simulink model "fc_KTH_lib"  (Simulink 4.00)
settings: Solver=FixedStepDiscrete  StartTime=0.0  StopTime=5  RelTol=1e-3
undefined symbols (not defined in the file or in its folder): cell_const_F, cell_const_g, cell_const_jo, cell_const_LHV_H2, cell_const_Mair, cell_const_MH, cell_const_MW, cell_const_R2, cell_const_Voc, fan_cool, fc_act, fc_blower_rec_H2, fc_blowera, fc_cell_const_eta1, fc_cell_const_eta_DCDC, fc_cell_const_etablow, fc_cell_const_etagen, fc_cell_const_etapump, fc_cell_const_ex, fc_cell_const_kw, fc_cell_const_Nrad, fc_cell_const_U, fc_cell_dim_A, fc_cell_dim_tm, fc_cell_press_a, fc_cell_press_amb, fc_cell_press_an, fc_cell_press_blowa, fc_cell_press_blowr, fc_cell_press_c, fc_cell_press_hum, fc_cell_press_hyd, fc_cell_stack_dpipe, fc_cell_stack_dpipefc, fc_cell_stack_drad, fc_cell_stack_Lpipe, fc_cell_stack_Lpipefc, fc_cell_stack_Lrad, fc_cell_stack_N, fc_cell_stack_Pel, fc_cell_stoich_RHah, fc_cell_stoich_RHch, fc_cell_stoich_RHo, fc_cell_stoich_vH, fc_cell_stoich_vO, fc_cell_stoich_XON, fc_cell_temp_ah, fc_cell_temp_amb, fc_cell_temp_cell, fc_cell_temp_ch, fc_cell_temp_cond, fc_cell_temp_cool, fc_cell_temp_evap, fc_cell_temp_rad, fc_cell_temp_ref, fc_compressor, fc_conda, fc_condc, fc_coolstack, fc_current ... (+10)
(part 2 of 2)

== system fc_KTH_lib/PEM fuel cell system/Subsystem1/Anode init/Saturation pressure  anode humidifier ==
  note: Saturation pressure of water in the anode humidifier
      | NOTE: [bar]
      | Data from "Anlaggnings- och apparatteknik", Westerlund, T., Abo Akademi, Finland, 1998
  Anode humidifier temperature [C] : Constant  Value=fc_cell_temp_ah
  Anode humidifier temperature [C]1 : Constant  Value=fc_cell_temp_ah
  Constant : Constant  Value=11.78
  Constant1 : Constant  Value=99.64
  Constant2 : Constant  Value=230
  Math Function : Math  Operator=exp  OutputSignalType=auto
  Product : Product  Inputs=*/  Multiplication=Element-wise(.*)  SaturateOnIntegerOverflow=on
  Product1 : Product  Inputs=2  Multiplication=Element-wise(.*)  SaturateOnIntegerOverflow=on
  Sum : Sum  Inputs=|+-  SaturateOnIntegerOverflow=on
  Sum1 : Sum  Inputs=|++  SaturateOnIntegerOverflow=on
  psatah : Outport  Port=1
  wires:
  Anode humidifier temperature [C]/1 -> Sum/1
  Constant1/1 -> Sum/2
  Anode humidifier temperature [C]1/1 -> Sum1/1
  Constant2/1 -> Sum1/2
  Sum/1 -> Product/1
  Sum1/1 -> Product/2
  Constant/1 -> Product1/2
  Product/1 -> Product1/1
  Product1/1 -> Math Function/1
  Math Function/1 -> psatah/1

== system fc_KTH_lib/PEM fuel cell system/Subsystem1/Anode init/Subsystem2 ==
  note: Activity of water vapor
  XWaI [-] : Inport  Port=1  LatchInput=off
  psatah [bar] : Inport  Port=2  LatchInput=off
  Anode pressure : Constant  Value=fc_cell_press_a
  Product : Product  Inputs=2  Multiplication=Element-wise(.*)  SaturateOnIntegerOverflow=on
  Product1 : Product  Inputs=*/  Multiplication=Element-wise(.*)  SaturateOnIntegerOverflow=on
  a : Outport  Port=1
  wires:
  XWaI [-]/1 -> Product/1
  Anode pressure/1 -> Product/2
  Product/1 -> Product1/1
  psatah [bar]/1 -> Product1/2
  Product1/1 -> a/1

== system fc_KTH_lib/PEM fuel cell system/Fuel cell stack, Heat Generation/Heat/Latent heat [W]/Heat of condensation ==
  note: Temperature in Celsius (C)
      | Tref=25 C
  note: 45.07E3 - 41.9*Tcell + 3.44E-3*Tcell^2 + 2.54E-6*Tcell^3 -8.98E-10*Tcell^4
  note: Heat of condensation [J/mol]
  Cell temperature [C] : Constant  Value=fc_cell_temp_cell
  Constant1 : Constant  Value=3.44E-3
  Constant2 : Constant  Value=45.07E3
  Constant3 : Constant  Value=41.9
  Constant4 : Constant  Value=2.54E-6
  Constant5 : Constant  Value=3
  Constant6 : Constant  Value=4
  Constant7 : Constant  Value=8.98E-10
  Math Function : Math  Operator=square  OutputSignalType=auto
  Math Function1 : Math  Operator=pow  OutputSignalType=auto
  Math Function2 : Math  Operator=pow  OutputSignalType=auto
  Product{,1..3} (4 alike) : Product  Inputs=2  Multiplication=Element-wise(.*)  SaturateOnIntegerOverflow=on
  Sum : Sum  Inputs=|++  SaturateOnIntegerOverflow=on
  Sum1 : Sum  Inputs=|+-  SaturateOnIntegerOverflow=on
  Sum2 : Sum  Inputs=|++  SaturateOnIntegerOverflow=on
  Sum3 : Sum  Inputs=|+-  SaturateOnIntegerOverflow=on
  Hcond [J/mol] : Outport  Port=1
  wires:
  Constant3/1 -> Product/1
  Cell temperature [C]/1 -> Product/2, Math Function/1, Math Function1/1, Math Function2/1
  Product1/1 -> Sum/2
  Product/1 -> Sum1/2
  Constant2/1 -> Sum1/1
  Sum1/1 -> Sum/1
  Sum/1 -> Sum2/1
  Constant1/1 -> Product1/1
  Math Function/1 -> Product1/2
  Math Function1/1 -> Product2/2
  Constant4/1 -> Product2/1
  Product2/1 -> Sum2/2
  Sum2/1 -> Sum3/1
  Sum3/1 -> Hcond [J/mol]/1
  Math Function2/1 -> Product3/2
  Product3/1 -> Sum3/2
  Constant7/1 -> Product3/1
  Constant5/1 -> Math Function1/2
  Constant6/1 -> Math Function2/2

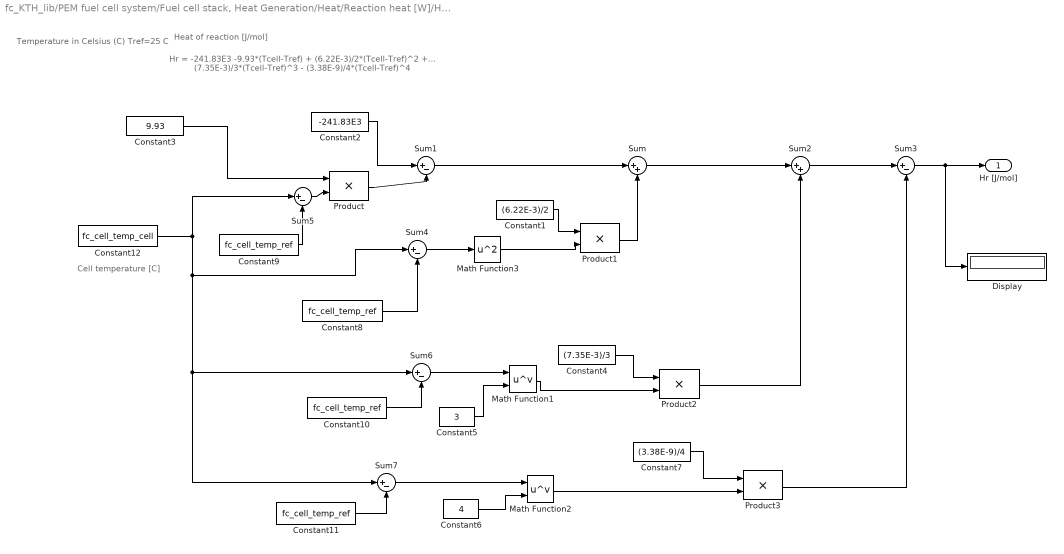
== system fc_KTH_lib/PEM fuel cell system/Fuel cell stack, Heat Generation/Heat/Reaction heat [W]/Heat of reaction ==
  note: Temperature in Celsius (C)
      | Tref=25 C
  note: Hr = -241.83E3 -9.93*(Tcell-Tref) + (6.22E-3)/2*(Tcell-Tref)^2 +...
      |   (7.35E-3)/3*(Tcell-Tref)^3 - (3.38E-9)/4*(Tcell-Tref)^4
  note: Heat of reaction [J/mol]
  note: Cell temperature [C]
  Constant1 : Constant  Value=(6.22E-3)/2
  Constant{8..11} (4 alike) : Constant  Value=fc_cell_temp_ref
  Constant12 : Constant  Value=fc_cell_temp_cell
  Constant2 : Constant  Value=-241.83E3
  Constant3 : Constant  Value=9.93
  Constant4 : Constant  Value=(7.35E-3)/3
  Constant5 : Constant  Value=3
  Constant6 : Constant  Value=4
  Constant7 : Constant  Value=(3.38E-9)/4
  Display : Display
      settings: Format=short  Decimation=12
  Math Function1 : Math  Operator=pow  OutputSignalType=auto
  Math Function2 : Math  Operator=pow  OutputSignalType=auto
  Math Function3 : Math  Operator=square  OutputSignalType=auto
  Product{,1..3} (4 alike) : Product  Inputs=2  Multiplication=Element-wise(.*)  SaturateOnIntegerOverflow=on
  Sum : Sum  Inputs=|++  SaturateOnIntegerOverflow=on
  Sum{1,3..7} (6 alike) : Sum  Inputs=|+-  SaturateOnIntegerOverflow=on
  Sum2 : Sum  Inputs=|++  SaturateOnIntegerOverflow=on
  Hr [J/mol] : Outport  Port=1
  wires:
  Constant3/1 -> Product/1
  Product1/1 -> Sum/2
  Product/1 -> Sum1/2
  Constant2/1 -> Sum1/1
  Sum1/1 -> Sum/1
  Sum/1 -> Sum2/1
  Constant1/1 -> Product1/1
  Math Function1/1 -> Product2/2
  Constant4/1 -> Product2/1
  Product2/1 -> Sum2/2
  Sum2/1 -> Sum3/1
  Sum3/1 -> Hr [J/mol]/1, Display/1
  Math Function2/1 -> Product3/2
  Product3/1 -> Sum3/2
  Constant7/1 -> Product3/1
  Constant5/1 -> Math Function1/2
  Constant6/1 -> Math Function2/2
  Constant8/1 -> Sum4/2
  Sum5/1 -> Product/2
  Constant9/1 -> Sum5/2
  Sum4/1 -> Math Function3/1
  Math Function3/1 -> Product1/2
  Constant10/1 -> Sum6/2
  Sum6/1 -> Math Function1/1
  Constant11/1 -> Sum7/2
  Sum7/1 -> Math Function2/1
  Constant12/1 -> Sum5/1, Sum4/1, Sum6/1, Sum7/1

== system fc_KTH_lib/PEM fuel cell system/Fuel cell stack, Heat Generation/Heat/Sensible heat [W]/Sensible heat in  ==
  note: Sensible heat in [W]
  note: Anode
  note: Cathode
  note: -------------------------------------------------------------------------------------------------------------------------------------------------------------------------------------------------------------------------------------------------------------------------------------------------------------------------------------------------------------------------------------------------------------------------------------------------------------------------------------------------------------------------------------------------------------------------------------------------------------------------------------------------------------------------------------------
  NinWa : Inport  Port=1  LatchInput=off
  NinHa : Inport  Port=2  LatchInput=off
  NinWc : Inport  Port=3  LatchInput=off
  NinO : Inport  Port=4  LatchInput=off
  NinN : Inport  Port=5  LatchInput=off
  "Enthalpy gaseous water, anode" : Subsystem
      settings: RTWFcnNameOpts=Auto  RTWFileNameOpts=Auto
  Enthalpy hydrogen in : Subsystem
      settings: RTWFcnNameOpts=Auto  RTWFileNameOpts=Auto
  Enthalpy nitrogen in : Subsystem
      settings: RTWFcnNameOpts=Auto  RTWFileNameOpts=Auto
  Enthalpy oxygen in : Subsystem
      settings: RTWFcnNameOpts=Auto  RTWFileNameOpts=Auto
  Product{,1..4} (5 alike) : Product  Inputs=2  Multiplication=Element-wise(.*)  SaturateOnIntegerOverflow=on
  Subsystem1 : Subsystem
      settings: RTWFcnNameOpts=Auto  RTWFileNameOpts=Auto
  Sum : Sum  Inputs=|++  SaturateOnIntegerOverflow=on
  Sum1 : Sum  Inputs=|++  SaturateOnIntegerOverflow=on
  Sum2 : Sum  Inputs=|++  SaturateOnIntegerOverflow=on
  sensina [W] : Outport  Port=1
  sensinc [W] : Outport  Port=2
  wires:
  NinHa/1 -> Product/1
  Enthalpy hydrogen in/1(h_Hin [J/mol]) -> Product/2
  Product/1 -> Sum/2
  NinWa/1 -> Product1/1
  Product1/1 -> Sum/1
  "Enthalpy gaseous water, anode"/1(h_Wgain [J/mol]) -> Product1/2
  NinWc/1 -> Product2/1
  Subsystem1/1(h_Wgcin [J/mol]) -> Product2/2
  Product2/1 -> Sum2/1
  NinO/1 -> Product3/1
  Enthalpy oxygen in/1(h_Oin [J/mol]) -> Product3/2
  Product3/1 -> Sum2/2
  Sum2/1 -> Sum1/1
  NinN/1 -> Product4/1
  Product4/1 -> Sum1/2
  Sum/1 -> sensina [W]/1
  Sum1/1 -> sensinc [W]/1
  Enthalpy nitrogen in/1(h_N [J/mol]) -> Product4/2

== system fc_KTH_lib/PEM fuel cell system/Fuel cell stack, Heat Generation/Heat/Sensible heat [W]/Sensible heat out ==
  note: Sensible heat out [W]
  note: Anode
  note: Cathode
  note: -------------------------------------------------------------------------------------------------------------------------------------------------------------------------------------------------------------------------------------------------------------------------------------------------------------------------------------------------------------------------------------------------------------------------------------------------------------------------------------------------------------------------------------------------------------------------------------------------------------------------------------------------------------------------------------------
  note: Enthalpy gaseous water, cathode
  NoutWag : Inport  Port=1  LatchInput=off
  NoutHa : Inport  Port=2  LatchInput=off
  NoutWcg : Inport  Port=3  LatchInput=off
  NoutO : Inport  Port=4  LatchInput=off
  NoutN : Inport  Port=5  LatchInput=off
  NoutWcl : Inport  Port=6  LatchInput=off
  "Enthalpy gaseous water, anode" : Subsystem
      settings: RTWFcnNameOpts=Auto  RTWFileNameOpts=Auto
  Enthalpy hydrogen in : Subsystem
      settings: RTWFcnNameOpts=Auto  RTWFileNameOpts=Auto
  Enthalpy nitrogen out : Subsystem
      settings: RTWFcnNameOpts=Auto  RTWFileNameOpts=Auto
  Enthalpy oxygen out : Subsystem
      settings: RTWFcnNameOpts=Auto  RTWFileNameOpts=Auto
  Product{,1..5} (6 alike) : Product  Inputs=2  Multiplication=Element-wise(.*)  SaturateOnIntegerOverflow=on
  Subsystem1 : Subsystem
      settings: RTWFcnNameOpts=Auto  RTWFileNameOpts=Auto
  Subsystem2 : Subsystem
      settings: RTWFcnNameOpts=Auto  RTWFileNameOpts=Auto
  Sum{,1..3} (4 alike) : Sum  Inputs=|++  SaturateOnIntegerOverflow=on
  sensouta [W] : Outport  Port=1
  sensoutc [W] : Outport  Port=2
  wires:
  NoutHa/1 -> Product/1
  Enthalpy hydrogen in/1(h_Hout [J/mol]) -> Product/2
  Product/1 -> Sum/2
  NoutWag/1 -> Product1/1
  Product1/1 -> Sum/1
  "Enthalpy gaseous water, anode"/1(h_Wgaout [J/mol]) -> Product1/2
  NoutWcg/1 -> Product2/1
  Subsystem1/1(h_Wgcout [J/mol]) -> Product2/2
  Product2/1 -> Sum2/1
  NoutO/1 -> Product3/1
  Enthalpy oxygen out/1(h_Oout [J/mol]) -> Product3/2
  Product3/1 -> Sum2/2
  Sum2/1 -> Sum1/1
  NoutN/1 -> Product4/1
  Product4/1 -> Sum1/2
  Sum/1 -> sensouta [W]/1
  Enthalpy nitrogen out/1(h_N [J/mol]) -> Product4/2
  Sum1/1 -> Sum3/1
  Sum3/1 -> sensoutc [W]/1
  Subsystem2/1(h_Wl [J/mol]) -> Product5/2
  Product5/1 -> Sum3/2
  NoutWcl/1 -> Product5/1

== system fc_KTH_lib/PEM fuel cell system/Humidifiers/Evapcooler/Ambient air/Humidity in air ==
  note: Humidity in air
  psat_air : Inport  Port=1  LatchInput=off
  Constant : Constant  Value=cell_const_MW
  Constant1 : Constant  Value=fc_cell_stoich_RHo
  Constant2 : Constant  Value=cell_const_Mair
  Constant3 : Constant  Value=fc_cell_press_amb
  Constant4 : Constant  Value=100
  Constant6 : Constant  Value=fc_cell_stoich_RHo
  Constant7 : Constant  Value=100
  Display : Display
      settings: Format=short
  Product : Product  Inputs=*/  Multiplication=Element-wise(.*)  SaturateOnIntegerOverflow=on
  Product1 : Product  Inputs=*/  Multiplication=Element-wise(.*)  SaturateOnIntegerOverflow=on
  Product2 : Product  Inputs=3  Multiplication=Element-wise(.*)  SaturateOnIntegerOverflow=on
  Product3 : Product  Inputs=*/  Multiplication=Element-wise(.*)  SaturateOnIntegerOverflow=on
  Product4 : Product  Inputs=2  Multiplication=Element-wise(.*)  SaturateOnIntegerOverflow=on
  Product5 : Product  Inputs=/*  Multiplication=Element-wise(.*)  SaturateOnIntegerOverflow=on
  Sum : Sum  Inputs=|+-  SaturateOnIntegerOverflow=on
  wires:
  Constant/1 -> Product/1
  Constant2/1 -> Product/2
  Constant1/1 -> Product1/1
  Constant4/1 -> Product1/2
  psat_air/1 -> Product2/1, Product4/2
  Product1/1 -> Product2/3
  Product/1 -> Product2/2
  Constant6/1 -> Product3/1
  Constant7/1 -> Product3/2
  Constant3/1 -> Sum/1
  Product3/1 -> Sum/2
  Sum/1 -> Product4/1
  Product2/1 -> Product5/2
  Product4/1 -> Product5/1
  Product5/1 -> Display/1

== system fc_KTH_lib/PEM fuel cell system/Humidifiers/Evapcooler/Ambient air/Saturation pressure ==
  note: Saturation pressure of water in the ambient air
      | NOTE: [bar]
      | Data from "Anlaggnings- och apparatteknik", Westerlund, T., Abo Akademi, Finland, 1998
  Ambient temperature [C] : Constant  Value=fc_cell_temp_amb
  Ambient temperature [C]1 : Constant  Value=fc_cell_temp_amb
  Constant : Constant  Value=11.78
  Constant1 : Constant  Value=99.64
  Constant2 : Constant  Value=230
  Math Function : Math  Operator=exp  OutputSignalType=auto
  Product : Product  Inputs=*/  Multiplication=Element-wise(.*)  SaturateOnIntegerOverflow=on
  Product1 : Product  Inputs=2  Multiplication=Element-wise(.*)  SaturateOnIntegerOverflow=on
  Sum : Sum  Inputs=|+-  SaturateOnIntegerOverflow=on
  Sum1 : Sum  Inputs=|++  SaturateOnIntegerOverflow=on
  psat_air : Outport  Port=1
  tag scope: psat_air=global
  wires:
  Ambient temperature [C]/1 -> Sum/1
  Constant1/1 -> Sum/2
  Ambient temperature [C]1/1 -> Sum1/1
  Constant2/1 -> Sum1/2
  Sum/1 -> Product/1
  Sum1/1 -> Product/2
  Constant/1 -> Product1/2
  Product/1 -> Product1/1
  Product1/1 -> Math Function/1
  Math Function/1 -> psat_air/1, [psat_air]

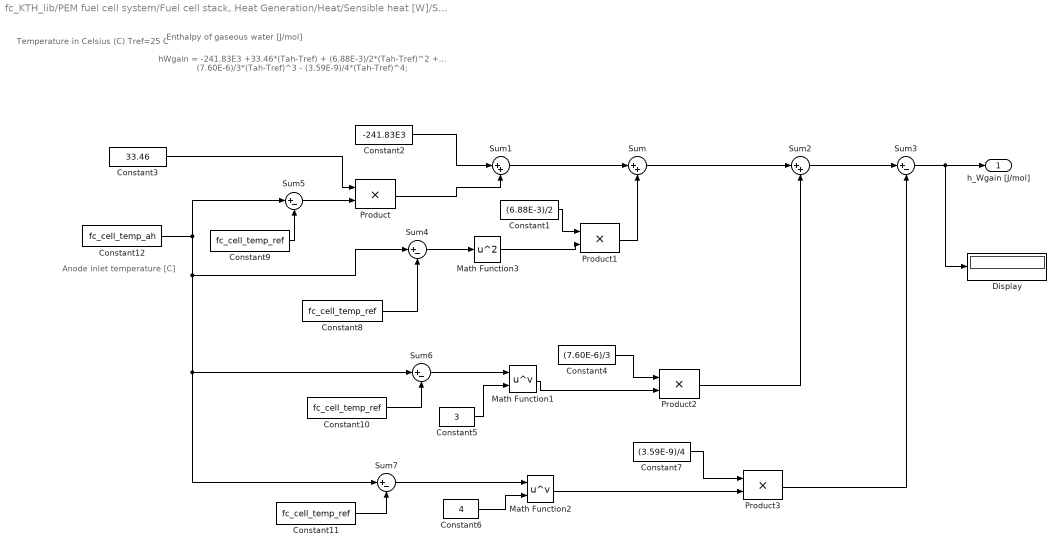
== system fc_KTH_lib/PEM fuel cell system/Fuel cell stack, Heat Generation/Heat/Sensible heat [W]/Sensible heat in /Enthalpy gaseous water, anode ==
  note: Temperature in Celsius (C)
      | Tref=25 C
  note: hWgain = -241.83E3 +33.46*(Tah-Tref) + (6.88E-3)/2*(Tah-Tref)^2 +...
      |    (7.60E-6)/3*(Tah-Tref)^3 - (3.59E-9)/4*(Tah-Tref)^4;
  note: Enthalpy of gaseous water [J/mol]
  note: Anode inlet temperature [C]
  Constant1 : Constant  Value=(6.88E-3)/2
  Constant{8..11} (4 alike) : Constant  Value=fc_cell_temp_ref
  Constant12 : Constant  Value=fc_cell_temp_ah
  Constant2 : Constant  Value=-241.83E3
  Constant3 : Constant  Value=33.46
  Constant4 : Constant  Value=(7.60E-6)/3
  Constant5 : Constant  Value=3
  Constant6 : Constant  Value=4
  Constant7 : Constant  Value=(3.59E-9)/4
  Display : Display
      settings: Format=short  Decimation=12
  Math Function1 : Math  Operator=pow  OutputSignalType=auto
  Math Function2 : Math  Operator=pow  OutputSignalType=auto
  Math Function3 : Math  Operator=square  OutputSignalType=auto
  Product{,1..3} (4 alike) : Product  Inputs=2  Multiplication=Element-wise(.*)  SaturateOnIntegerOverflow=on
  Sum : Sum  Inputs=|++  SaturateOnIntegerOverflow=on
  Sum1 : Sum  Inputs=|++  SaturateOnIntegerOverflow=on
  Sum2 : Sum  Inputs=|++  SaturateOnIntegerOverflow=on
  Sum{3..7} (5 alike) : Sum  Inputs=|+-  SaturateOnIntegerOverflow=on
  h_Wgain [J/mol] : Outport  Port=1
  wires:
  Constant3/1 -> Product/1
  Product1/1 -> Sum/2
  Sum/1 -> Sum2/1
  Constant1/1 -> Product1/1
  Math Function1/1 -> Product2/2
  Constant4/1 -> Product2/1
  Product2/1 -> Sum2/2
  Sum2/1 -> Sum3/1
  Sum3/1 -> h_Wgain [J/mol]/1, Display/1
  Math Function2/1 -> Product3/2
  Product3/1 -> Sum3/2
  Constant7/1 -> Product3/1
  Constant5/1 -> Math Function1/2
  Constant6/1 -> Math Function2/2
  Constant8/1 -> Sum4/2
  Sum5/1 -> Product/2
  Constant9/1 -> Sum5/2
  Sum4/1 -> Math Function3/1
  Math Function3/1 -> Product1/2
  Constant10/1 -> Sum6/2
  Sum6/1 -> Math Function1/1
  Constant11/1 -> Sum7/2
  Sum7/1 -> Math Function2/1
  Constant12/1 -> Sum5/1, Sum4/1, Sum6/1, Sum7/1
  Product/1 -> Sum1/2
  Sum1/1 -> Sum/1
  Constant2/1 -> Sum1/1

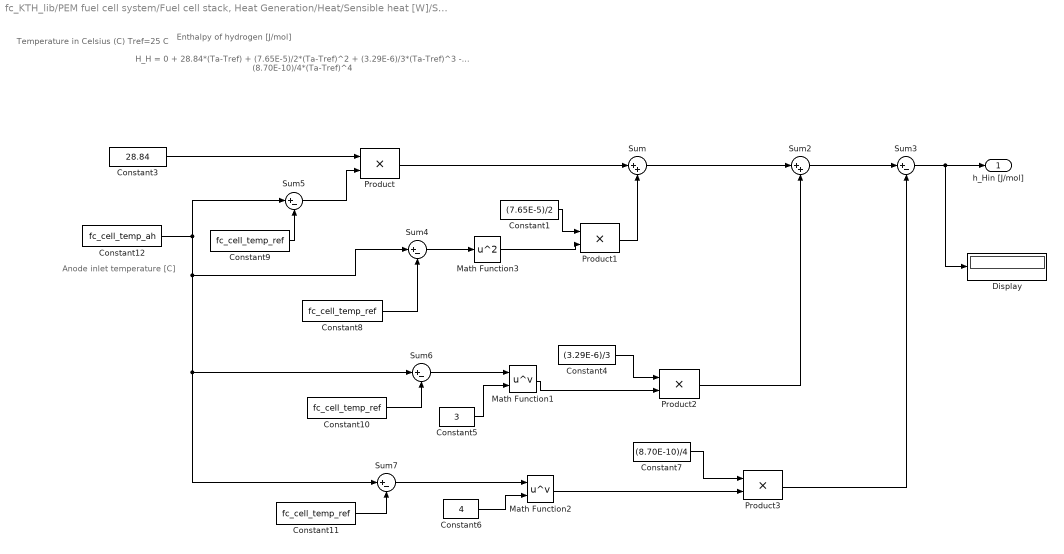
== system fc_KTH_lib/PEM fuel cell system/Fuel cell stack, Heat Generation/Heat/Sensible heat [W]/Sensible heat in /Enthalpy hydrogen in ==
  note: Temperature in Celsius (C)
      | Tref=25 C
  note: H_H = 0 + 28.84*(Ta-Tref) + (7.65E-5)/2*(Ta-Tref)^2 + (3.29E-6)/3*(Ta-Tref)^3 -...
      |    (8.70E-10)/4*(Ta-Tref)^4
  note: Enthalpy of hydrogen [J/mol]
  note: Anode inlet temperature [C]
  Constant1 : Constant  Value=(7.65E-5)/2
  Constant{8..11} (4 alike) : Constant  Value=fc_cell_temp_ref
  Constant12 : Constant  Value=fc_cell_temp_ah
  Constant3 : Constant  Value=28.84
  Constant4 : Constant  Value=(3.29E-6)/3
  Constant5 : Constant  Value=3
  Constant6 : Constant  Value=4
  Constant7 : Constant  Value=(8.70E-10)/4
  Display : Display
      settings: Format=short  Decimation=12
  Math Function1 : Math  Operator=pow  OutputSignalType=auto
  Math Function2 : Math  Operator=pow  OutputSignalType=auto
  Math Function3 : Math  Operator=square  OutputSignalType=auto
  Product{,1..3} (4 alike) : Product  Inputs=2  Multiplication=Element-wise(.*)  SaturateOnIntegerOverflow=on
  Sum : Sum  Inputs=|++  SaturateOnIntegerOverflow=on
  Sum2 : Sum  Inputs=|++  SaturateOnIntegerOverflow=on
  Sum{3..7} (5 alike) : Sum  Inputs=|+-  SaturateOnIntegerOverflow=on
  h_Hin [J/mol] : Outport  Port=1
  wires:
  Constant3/1 -> Product/1
  Product1/1 -> Sum/2
  Sum/1 -> Sum2/1
  Constant1/1 -> Product1/1
  Math Function1/1 -> Product2/2
  Constant4/1 -> Product2/1
  Product2/1 -> Sum2/2
  Sum2/1 -> Sum3/1
  Sum3/1 -> h_Hin [J/mol]/1, Display/1
  Math Function2/1 -> Product3/2
  Product3/1 -> Sum3/2
  Constant7/1 -> Product3/1
  Constant5/1 -> Math Function1/2
  Constant6/1 -> Math Function2/2
  Constant8/1 -> Sum4/2
  Sum5/1 -> Product/2
  Constant9/1 -> Sum5/2
  Sum4/1 -> Math Function3/1
  Math Function3/1 -> Product1/2
  Constant10/1 -> Sum6/2
  Sum6/1 -> Math Function1/1
  Constant11/1 -> Sum7/2
  Sum7/1 -> Math Function2/1
  Constant12/1 -> Sum5/1, Sum4/1, Sum6/1, Sum7/1
  Product/1 -> Sum/1

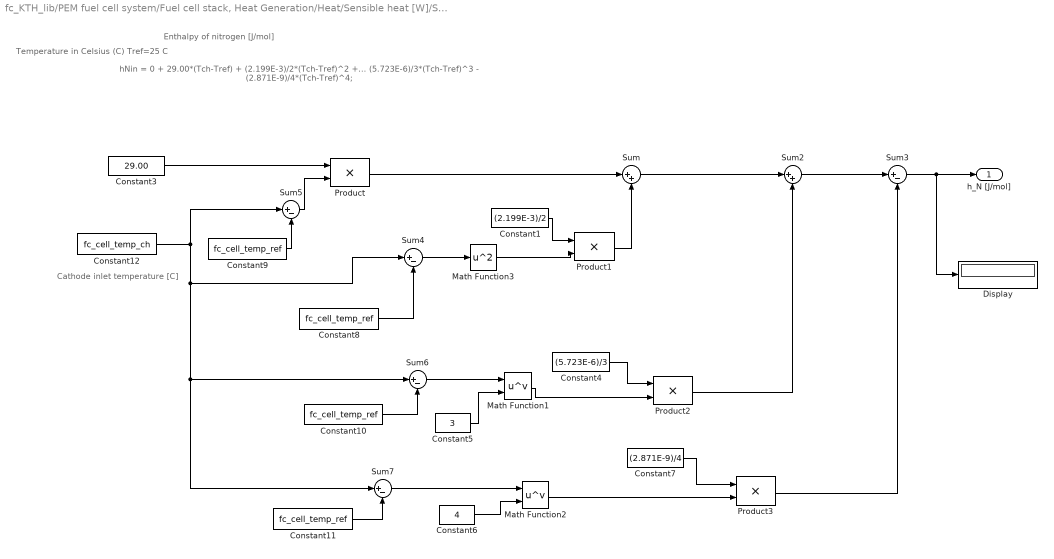
== system fc_KTH_lib/PEM fuel cell system/Fuel cell stack, Heat Generation/Heat/Sensible heat [W]/Sensible heat in /Enthalpy nitrogen in ==
  note: Temperature in Celsius (C)
      | Tref=25 C
  note: hNin = 0 + 29.00*(Tch-Tref) + (2.199E-3)/2*(Tch-Tref)^2 +...
      |    (5.723E-6)/3*(Tch-Tref)^3 - (2.871E-9)/4*(Tch-Tref)^4;
  note: Enthalpy of nitrogen [J/mol]
  note: Cathode inlet temperature [C]
  Constant1 : Constant  Value=(2.199E-3)/2
  Constant{8..11} (4 alike) : Constant  Value=fc_cell_temp_ref
  Constant12 : Constant  Value=fc_cell_temp_ch
  Constant3 : Constant  Value=29.00
  Constant4 : Constant  Value=(5.723E-6)/3
  Constant5 : Constant  Value=3
  Constant6 : Constant  Value=4
  Constant7 : Constant  Value=(2.871E-9)/4
  Display : Display
      settings: Format=short  Decimation=12
  Math Function1 : Math  Operator=pow  OutputSignalType=auto
  Math Function2 : Math  Operator=pow  OutputSignalType=auto
  Math Function3 : Math  Operator=square  OutputSignalType=auto
  Product{,1..3} (4 alike) : Product  Inputs=2  Multiplication=Element-wise(.*)  SaturateOnIntegerOverflow=on
  Sum : Sum  Inputs=|++  SaturateOnIntegerOverflow=on
  Sum2 : Sum  Inputs=|++  SaturateOnIntegerOverflow=on
  Sum{3..7} (5 alike) : Sum  Inputs=|+-  SaturateOnIntegerOverflow=on
  h_N [J/mol] : Outport  Port=1
  wires:
  Constant3/1 -> Product/1
  Product1/1 -> Sum/2
  Product/1 -> Sum/1
  Sum/1 -> Sum2/1
  Constant1/1 -> Product1/1
  Math Function1/1 -> Product2/2
  Constant4/1 -> Product2/1
  Product2/1 -> Sum2/2
  Sum2/1 -> Sum3/1
  Sum3/1 -> h_N [J/mol]/1, Display/1
  Math Function2/1 -> Product3/2
  Product3/1 -> Sum3/2
  Constant7/1 -> Product3/1
  Constant5/1 -> Math Function1/2
  Constant6/1 -> Math Function2/2
  Constant8/1 -> Sum4/2
  Sum5/1 -> Product/2
  Constant9/1 -> Sum5/2
  Sum4/1 -> Math Function3/1
  Math Function3/1 -> Product1/2
  Constant10/1 -> Sum6/2
  Sum6/1 -> Math Function1/1
  Constant11/1 -> Sum7/2
  Sum7/1 -> Math Function2/1
  Constant12/1 -> Sum5/1, Sum4/1, Sum6/1, Sum7/1

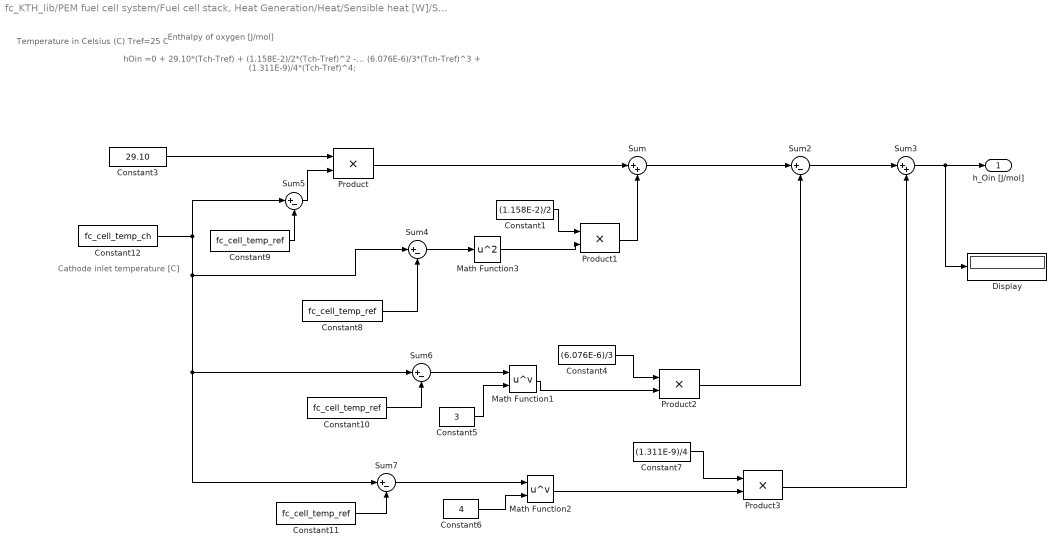
== system fc_KTH_lib/PEM fuel cell system/Fuel cell stack, Heat Generation/Heat/Sensible heat [W]/Sensible heat in /Enthalpy oxygen in ==
  note: Temperature in Celsius (C)
      | Tref=25 C
  note: hOin =0 + 29.10*(Tch-Tref) + (1.158E-2)/2*(Tch-Tref)^2 -...
      |    (6.076E-6)/3*(Tch-Tref)^3 + (1.311E-9)/4*(Tch-Tref)^4;
  note: Enthalpy of oxygen [J/mol]
  note: Cathode inlet temperature [C]
  Constant1 : Constant  Value=(1.158E-2)/2
  Constant{8..11} (4 alike) : Constant  Value=fc_cell_temp_ref
  Constant12 : Constant  Value=fc_cell_temp_ch
  Constant3 : Constant  Value=29.10
  Constant4 : Constant  Value=(6.076E-6)/3
  Constant5 : Constant  Value=3
  Constant6 : Constant  Value=4
  Constant7 : Constant  Value=(1.311E-9)/4
  Display : Display
      settings: Format=short  Decimation=12
  Math Function1 : Math  Operator=pow  OutputSignalType=auto
  Math Function2 : Math  Operator=pow  OutputSignalType=auto
  Math Function3 : Math  Operator=square  OutputSignalType=auto
  Product{,1..3} (4 alike) : Product  Inputs=2  Multiplication=Element-wise(.*)  SaturateOnIntegerOverflow=on
  Sum : Sum  Inputs=|++  SaturateOnIntegerOverflow=on
  Sum{2,4..7} (5 alike) : Sum  Inputs=|+-  SaturateOnIntegerOverflow=on
  Sum3 : Sum  Inputs=|++  SaturateOnIntegerOverflow=on
  h_Oin [J/mol] : Outport  Port=1
  wires:
  Constant3/1 -> Product/1
  Product1/1 -> Sum/2
  Product/1 -> Sum/1
  Sum/1 -> Sum2/1
  Constant1/1 -> Product1/1
  Math Function1/1 -> Product2/2
  Constant4/1 -> Product2/1
  Product2/1 -> Sum2/2
  Sum2/1 -> Sum3/1
  Sum3/1 -> h_Oin [J/mol]/1, Display/1
  Math Function2/1 -> Product3/2
  Product3/1 -> Sum3/2
  Constant7/1 -> Product3/1
  Constant5/1 -> Math Function1/2
  Constant6/1 -> Math Function2/2
  Constant8/1 -> Sum4/2
  Sum5/1 -> Product/2
  Constant9/1 -> Sum5/2
  Sum4/1 -> Math Function3/1
  Math Function3/1 -> Product1/2
  Constant10/1 -> Sum6/2
  Sum6/1 -> Math Function1/1
  Constant11/1 -> Sum7/2
  Sum7/1 -> Math Function2/1
  Constant12/1 -> Sum5/1, Sum4/1, Sum6/1, Sum7/1

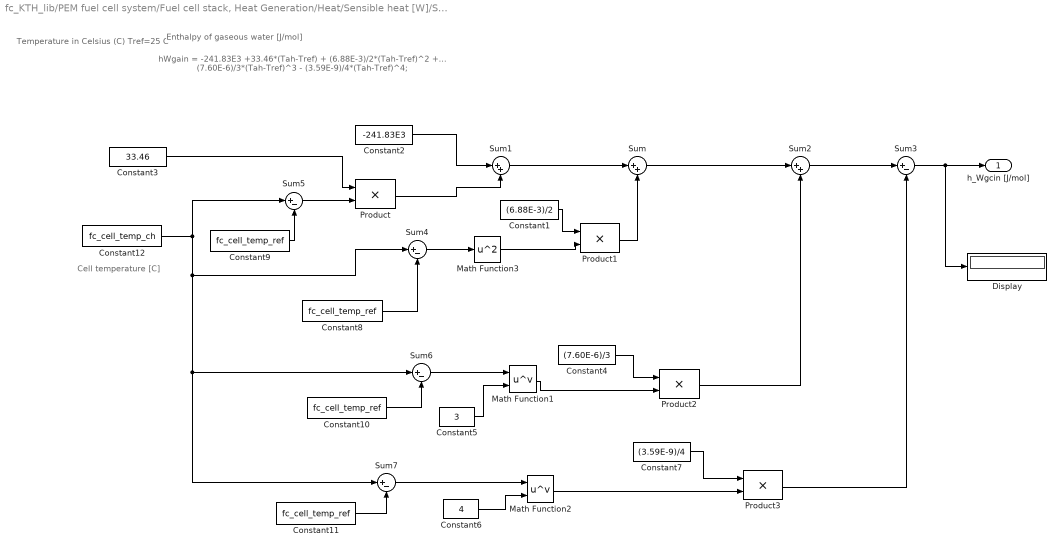
== system fc_KTH_lib/PEM fuel cell system/Fuel cell stack, Heat Generation/Heat/Sensible heat [W]/Sensible heat in /Subsystem1 ==
  note: Temperature in Celsius (C)
      | Tref=25 C
  note: hWgain = -241.83E3 +33.46*(Tah-Tref) + (6.88E-3)/2*(Tah-Tref)^2 +...
      |    (7.60E-6)/3*(Tah-Tref)^3 - (3.59E-9)/4*(Tah-Tref)^4;
  note: Enthalpy of gaseous water [J/mol]
  note: Cell temperature [C]
  Constant1 : Constant  Value=(6.88E-3)/2
  Constant{8..11} (4 alike) : Constant  Value=fc_cell_temp_ref
  Constant12 : Constant  Value=fc_cell_temp_ch
  Constant2 : Constant  Value=-241.83E3
  Constant3 : Constant  Value=33.46
  Constant4 : Constant  Value=(7.60E-6)/3
  Constant5 : Constant  Value=3
  Constant6 : Constant  Value=4
  Constant7 : Constant  Value=(3.59E-9)/4
  Display : Display
      settings: Format=short  Decimation=12
  Math Function1 : Math  Operator=pow  OutputSignalType=auto
  Math Function2 : Math  Operator=pow  OutputSignalType=auto
  Math Function3 : Math  Operator=square  OutputSignalType=auto
  Product{,1..3} (4 alike) : Product  Inputs=2  Multiplication=Element-wise(.*)  SaturateOnIntegerOverflow=on
  Sum : Sum  Inputs=|++  SaturateOnIntegerOverflow=on
  Sum1 : Sum  Inputs=|++  SaturateOnIntegerOverflow=on
  Sum2 : Sum  Inputs=|++  SaturateOnIntegerOverflow=on
  Sum{3..7} (5 alike) : Sum  Inputs=|+-  SaturateOnIntegerOverflow=on
  h_Wgcin [J/mol] : Outport  Port=1
  wires:
  Constant3/1 -> Product/1
  Product1/1 -> Sum/2
  Sum/1 -> Sum2/1
  Constant1/1 -> Product1/1
  Math Function1/1 -> Product2/2
  Constant4/1 -> Product2/1
  Product2/1 -> Sum2/2
  Sum2/1 -> Sum3/1
  Sum3/1 -> h_Wgcin [J/mol]/1, Display/1
  Math Function2/1 -> Product3/2
  Product3/1 -> Sum3/2
  Constant7/1 -> Product3/1
  Constant5/1 -> Math Function1/2
  Constant6/1 -> Math Function2/2
  Constant8/1 -> Sum4/2
  Sum5/1 -> Product/2
  Constant9/1 -> Sum5/2
  Sum4/1 -> Math Function3/1
  Math Function3/1 -> Product1/2
  Constant10/1 -> Sum6/2
  Sum6/1 -> Math Function1/1
  Constant11/1 -> Sum7/2
  Sum7/1 -> Math Function2/1
  Constant12/1 -> Sum5/1, Sum4/1, Sum6/1, Sum7/1
  Product/1 -> Sum1/2
  Sum1/1 -> Sum/1
  Constant2/1 -> Sum1/1

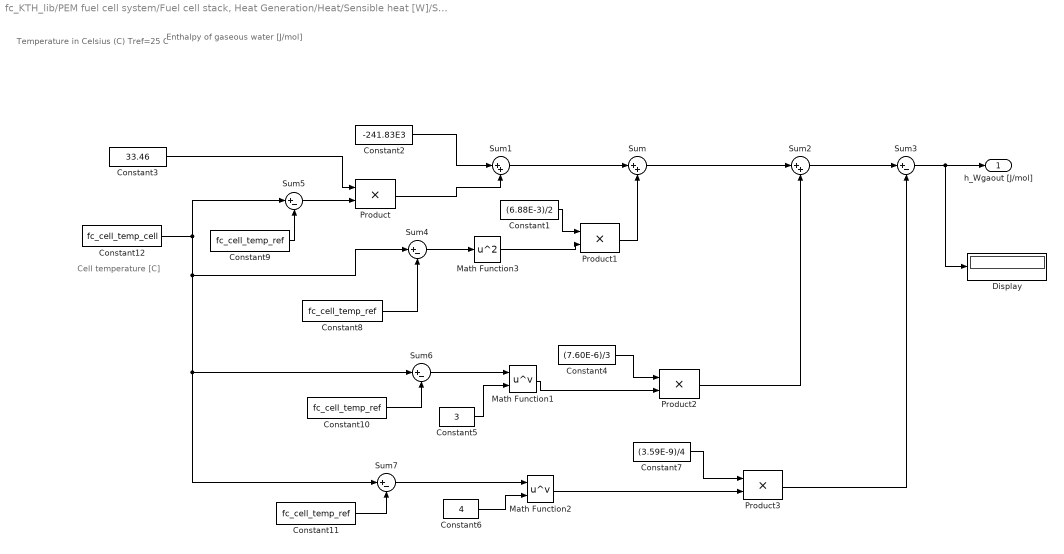
== system fc_KTH_lib/PEM fuel cell system/Fuel cell stack, Heat Generation/Heat/Sensible heat [W]/Sensible heat out/Enthalpy gaseous water, anode ==
  note: Temperature in Celsius (C)
      | Tref=25 C
  note: Enthalpy of gaseous water [J/mol]
  note: Cell temperature [C]
  Constant1 : Constant  Value=(6.88E-3)/2
  Constant{8..11} (4 alike) : Constant  Value=fc_cell_temp_ref
  Constant12 : Constant  Value=fc_cell_temp_cell
  Constant2 : Constant  Value=-241.83E3
  Constant3 : Constant  Value=33.46
  Constant4 : Constant  Value=(7.60E-6)/3
  Constant5 : Constant  Value=3
  Constant6 : Constant  Value=4
  Constant7 : Constant  Value=(3.59E-9)/4
  Display : Display
      settings: Format=short  Decimation=12
  Math Function1 : Math  Operator=pow  OutputSignalType=auto
  Math Function2 : Math  Operator=pow  OutputSignalType=auto
  Math Function3 : Math  Operator=square  OutputSignalType=auto
  Product{,1..3} (4 alike) : Product  Inputs=2  Multiplication=Element-wise(.*)  SaturateOnIntegerOverflow=on
  Sum : Sum  Inputs=|++  SaturateOnIntegerOverflow=on
  Sum1 : Sum  Inputs=|++  SaturateOnIntegerOverflow=on
  Sum2 : Sum  Inputs=|++  SaturateOnIntegerOverflow=on
  Sum{3..7} (5 alike) : Sum  Inputs=|+-  SaturateOnIntegerOverflow=on
  h_Wgaout [J/mol] : Outport  Port=1
  wires:
  Constant3/1 -> Product/1
  Product1/1 -> Sum/2
  Sum/1 -> Sum2/1
  Constant1/1 -> Product1/1
  Math Function1/1 -> Product2/2
  Constant4/1 -> Product2/1
  Product2/1 -> Sum2/2
  Sum2/1 -> Sum3/1
  Sum3/1 -> h_Wgaout [J/mol]/1, Display/1
  Math Function2/1 -> Product3/2
  Product3/1 -> Sum3/2
  Constant7/1 -> Product3/1
  Constant5/1 -> Math Function1/2
  Constant6/1 -> Math Function2/2
  Constant8/1 -> Sum4/2
  Sum5/1 -> Product/2
  Constant9/1 -> Sum5/2
  Sum4/1 -> Math Function3/1
  Math Function3/1 -> Product1/2
  Constant10/1 -> Sum6/2
  Sum6/1 -> Math Function1/1
  Constant11/1 -> Sum7/2
  Sum7/1 -> Math Function2/1
  Constant12/1 -> Sum5/1, Sum4/1, Sum6/1, Sum7/1
  Product/1 -> Sum1/2
  Sum1/1 -> Sum/1
  Constant2/1 -> Sum1/1

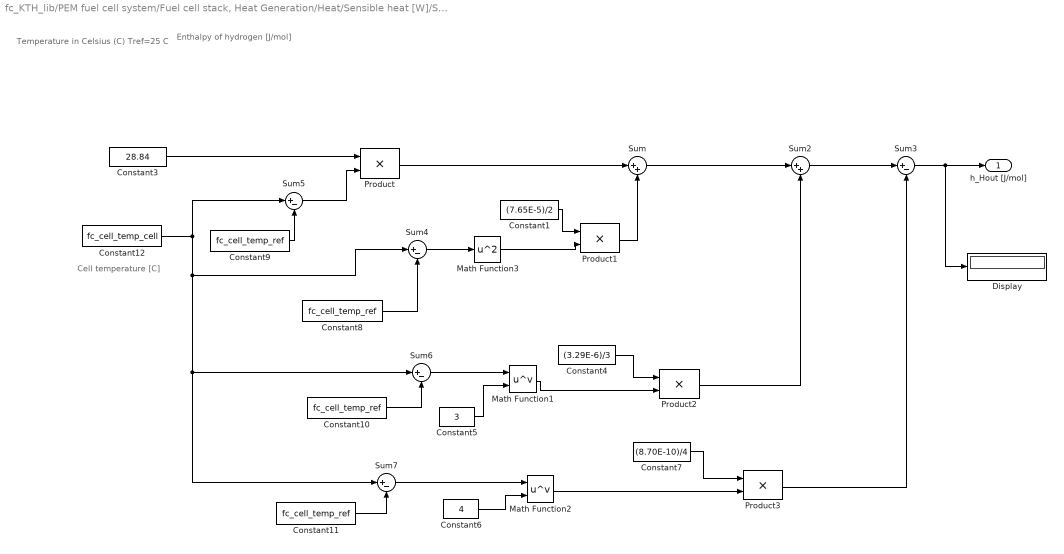
== system fc_KTH_lib/PEM fuel cell system/Fuel cell stack, Heat Generation/Heat/Sensible heat [W]/Sensible heat out/Enthalpy hydrogen in ==
  note: Temperature in Celsius (C)
      | Tref=25 C
  note: Enthalpy of hydrogen [J/mol]
  note: Cell temperature [C]
  Constant1 : Constant  Value=(7.65E-5)/2
  Constant{8..11} (4 alike) : Constant  Value=fc_cell_temp_ref
  Constant12 : Constant  Value=fc_cell_temp_cell
  Constant3 : Constant  Value=28.84
  Constant4 : Constant  Value=(3.29E-6)/3
  Constant5 : Constant  Value=3
  Constant6 : Constant  Value=4
  Constant7 : Constant  Value=(8.70E-10)/4
  Display : Display
      settings: Format=short  Decimation=12
  Math Function1 : Math  Operator=pow  OutputSignalType=auto
  Math Function2 : Math  Operator=pow  OutputSignalType=auto
  Math Function3 : Math  Operator=square  OutputSignalType=auto
  Product{,1..3} (4 alike) : Product  Inputs=2  Multiplication=Element-wise(.*)  SaturateOnIntegerOverflow=on
  Sum : Sum  Inputs=|++  SaturateOnIntegerOverflow=on
  Sum2 : Sum  Inputs=|++  SaturateOnIntegerOverflow=on
  Sum{3..7} (5 alike) : Sum  Inputs=|+-  SaturateOnIntegerOverflow=on
  h_Hout [J/mol] : Outport  Port=1
  wires:
  Constant3/1 -> Product/1
  Product1/1 -> Sum/2
  Sum/1 -> Sum2/1
  Constant1/1 -> Product1/1
  Math Function1/1 -> Product2/2
  Constant4/1 -> Product2/1
  Product2/1 -> Sum2/2
  Sum2/1 -> Sum3/1
  Sum3/1 -> h_Hout [J/mol]/1, Display/1
  Math Function2/1 -> Product3/2
  Product3/1 -> Sum3/2
  Constant7/1 -> Product3/1
  Constant5/1 -> Math Function1/2
  Constant6/1 -> Math Function2/2
  Constant8/1 -> Sum4/2
  Sum5/1 -> Product/2
  Constant9/1 -> Sum5/2
  Sum4/1 -> Math Function3/1
  Math Function3/1 -> Product1/2
  Constant10/1 -> Sum6/2
  Sum6/1 -> Math Function1/1
  Constant11/1 -> Sum7/2
  Sum7/1 -> Math Function2/1
  Constant12/1 -> Sum5/1, Sum4/1, Sum6/1, Sum7/1
  Product/1 -> Sum/1

== system fc_KTH_lib/PEM fuel cell system/Fuel cell stack, Heat Generation/Heat/Sensible heat [W]/Sensible heat out/Enthalpy nitrogen out ==
  note: Temperature in Celsius (C)
      | Tref=25 C
  note: Enthalpy of nitrogen [J/mol]
  note: Cell temperature [C]
  Constant1 : Constant  Value=(2.199E-3)/2
  Constant{8..11} (4 alike) : Constant  Value=fc_cell_temp_ref
  Constant12 : Constant  Value=fc_cell_temp_cell
  Constant3 : Constant  Value=29.00
  Constant4 : Constant  Value=(5.723E-6)/3
  Constant5 : Constant  Value=3
  Constant6 : Constant  Value=4
  Constant7 : Constant  Value=(2.871E-9)/4
  Display : Display
      settings: Format=short  Decimation=12
  Math Function1 : Math  Operator=pow  OutputSignalType=auto
  Math Function2 : Math  Operator=pow  OutputSignalType=auto
  Math Function3 : Math  Operator=square  OutputSignalType=auto
  Product{,1..3} (4 alike) : Product  Inputs=2  Multiplication=Element-wise(.*)  SaturateOnIntegerOverflow=on
  Sum : Sum  Inputs=|++  SaturateOnIntegerOverflow=on
  Sum2 : Sum  Inputs=|++  SaturateOnIntegerOverflow=on
  Sum{3..7} (5 alike) : Sum  Inputs=|+-  SaturateOnIntegerOverflow=on
  h_N [J/mol] : Outport  Port=1
  wires:
  Constant3/1 -> Product/1
  Product1/1 -> Sum/2
  Product/1 -> Sum/1
  Sum/1 -> Sum2/1
  Constant1/1 -> Product1/1
  Math Function1/1 -> Product2/2
  Constant4/1 -> Product2/1
  Product2/1 -> Sum2/2
  Sum2/1 -> Sum3/1
  Sum3/1 -> h_N [J/mol]/1, Display/1
  Math Function2/1 -> Product3/2
  Product3/1 -> Sum3/2
  Constant7/1 -> Product3/1
  Constant5/1 -> Math Function1/2
  Constant6/1 -> Math Function2/2
  Constant8/1 -> Sum4/2
  Sum5/1 -> Product/2
  Constant9/1 -> Sum5/2
  Sum4/1 -> Math Function3/1
  Math Function3/1 -> Product1/2
  Constant10/1 -> Sum6/2
  Sum6/1 -> Math Function1/1
  Constant11/1 -> Sum7/2
  Sum7/1 -> Math Function2/1
  Constant12/1 -> Sum5/1, Sum4/1, Sum6/1, Sum7/1

== system fc_KTH_lib/PEM fuel cell system/Fuel cell stack, Heat Generation/Heat/Sensible heat [W]/Sensible heat out/Enthalpy oxygen out ==
  note: Temperature in Celsius (C)
      | Tref=25 C
  note: Enthalpy of oxygen [J/mol]
  note: Cell temperature [C]
  Constant1 : Constant  Value=(1.158E-2)/2
  Constant{8..11} (4 alike) : Constant  Value=fc_cell_temp_ref
  Constant12 : Constant  Value=fc_cell_temp_cell
  Constant3 : Constant  Value=29.10
  Constant4 : Constant  Value=(6.076E-6)/3
  Constant5 : Constant  Value=3
  Constant6 : Constant  Value=4
  Constant7 : Constant  Value=(1.311E-9)/4
  Display : Display
      settings: Format=short  Decimation=12
  Math Function1 : Math  Operator=pow  OutputSignalType=auto
  Math Function2 : Math  Operator=pow  OutputSignalType=auto
  Math Function3 : Math  Operator=square  OutputSignalType=auto
  Product{,1..3} (4 alike) : Product  Inputs=2  Multiplication=Element-wise(.*)  SaturateOnIntegerOverflow=on
  Sum : Sum  Inputs=|++  SaturateOnIntegerOverflow=on
  Sum{2,4..7} (5 alike) : Sum  Inputs=|+-  SaturateOnIntegerOverflow=on
  Sum3 : Sum  Inputs=|++  SaturateOnIntegerOverflow=on
  h_Oout [J/mol] : Outport  Port=1
  wires:
  Constant3/1 -> Product/1
  Product1/1 -> Sum/2
  Product/1 -> Sum/1
  Sum/1 -> Sum2/1
  Constant1/1 -> Product1/1
  Math Function1/1 -> Product2/2
  Constant4/1 -> Product2/1
  Product2/1 -> Sum2/2
  Sum2/1 -> Sum3/1
  Sum3/1 -> h_Oout [J/mol]/1, Display/1
  Math Function2/1 -> Product3/2
  Product3/1 -> Sum3/2
  Constant7/1 -> Product3/1
  Constant5/1 -> Math Function1/2
  Constant6/1 -> Math Function2/2
  Constant8/1 -> Sum4/2
  Sum5/1 -> Product/2
  Constant9/1 -> Sum5/2
  Sum4/1 -> Math Function3/1
  Math Function3/1 -> Product1/2
  Constant10/1 -> Sum6/2
  Sum6/1 -> Math Function1/1
  Constant11/1 -> Sum7/2
  Sum7/1 -> Math Function2/1
  Constant12/1 -> Sum5/1, Sum4/1, Sum6/1, Sum7/1

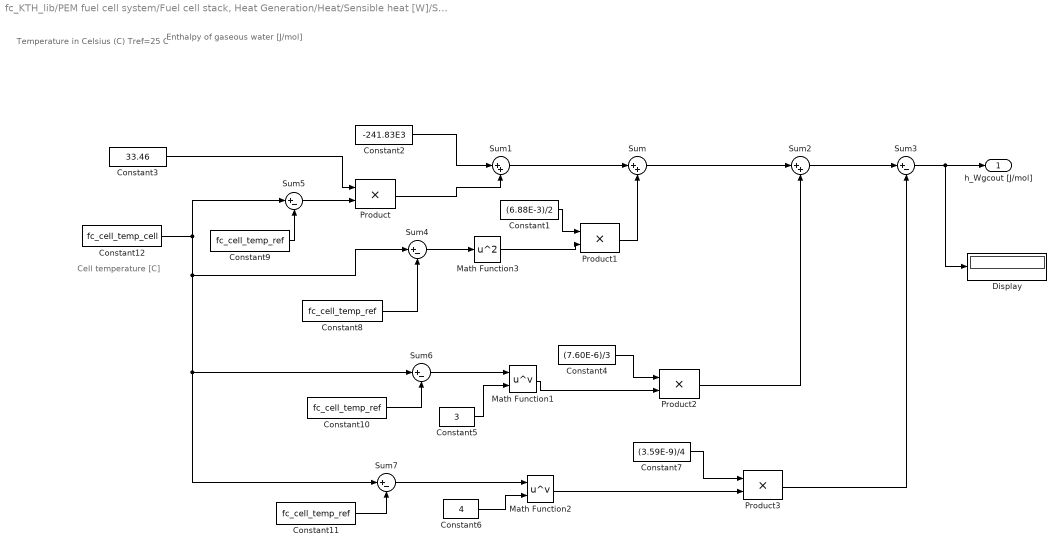
== system fc_KTH_lib/PEM fuel cell system/Fuel cell stack, Heat Generation/Heat/Sensible heat [W]/Sensible heat out/Subsystem1 ==
  note: Temperature in Celsius (C)
      | Tref=25 C
  note: Enthalpy of gaseous water [J/mol]
  note: Cell temperature [C]
  Constant1 : Constant  Value=(6.88E-3)/2
  Constant{8..11} (4 alike) : Constant  Value=fc_cell_temp_ref
  Constant12 : Constant  Value=fc_cell_temp_cell
  Constant2 : Constant  Value=-241.83E3
  Constant3 : Constant  Value=33.46
  Constant4 : Constant  Value=(7.60E-6)/3
  Constant5 : Constant  Value=3
  Constant6 : Constant  Value=4
  Constant7 : Constant  Value=(3.59E-9)/4
  Display : Display
      settings: Format=short  Decimation=12
  Math Function1 : Math  Operator=pow  OutputSignalType=auto
  Math Function2 : Math  Operator=pow  OutputSignalType=auto
  Math Function3 : Math  Operator=square  OutputSignalType=auto
  Product{,1..3} (4 alike) : Product  Inputs=2  Multiplication=Element-wise(.*)  SaturateOnIntegerOverflow=on
  Sum : Sum  Inputs=|++  SaturateOnIntegerOverflow=on
  Sum1 : Sum  Inputs=|++  SaturateOnIntegerOverflow=on
  Sum2 : Sum  Inputs=|++  SaturateOnIntegerOverflow=on
  Sum{3..7} (5 alike) : Sum  Inputs=|+-  SaturateOnIntegerOverflow=on
  h_Wgcout [J/mol] : Outport  Port=1
  wires:
  Constant3/1 -> Product/1
  Product1/1 -> Sum/2
  Sum/1 -> Sum2/1
  Constant1/1 -> Product1/1
  Math Function1/1 -> Product2/2
  Constant4/1 -> Product2/1
  Product2/1 -> Sum2/2
  Sum2/1 -> Sum3/1
  Sum3/1 -> h_Wgcout [J/mol]/1, Display/1
  Math Function2/1 -> Product3/2
  Product3/1 -> Sum3/2
  Constant7/1 -> Product3/1
  Constant5/1 -> Math Function1/2
  Constant6/1 -> Math Function2/2
  Constant8/1 -> Sum4/2
  Sum5/1 -> Product/2
  Constant9/1 -> Sum5/2
  Sum4/1 -> Math Function3/1
  Math Function3/1 -> Product1/2
  Constant10/1 -> Sum6/2
  Sum6/1 -> Math Function1/1
  Constant11/1 -> Sum7/2
  Sum7/1 -> Math Function2/1
  Constant12/1 -> Sum5/1, Sum4/1, Sum6/1, Sum7/1
  Product/1 -> Sum1/2
  Sum1/1 -> Sum/1
  Constant2/1 -> Sum1/1

== system fc_KTH_lib/PEM fuel cell system/Fuel cell stack, Heat Generation/Heat/Sensible heat [W]/Sensible heat out/Subsystem2 ==
  note: Temperature in Celsius (C)
      | Tref=25 C
  note: HWl = -285.84E3 + 75.38*(Tcell-Tref)
  note: Enthalpy of liquid water [J/mol]
  note: Cell temperature [C]
  Constant12 : Constant  Value=fc_cell_temp_cell
  Constant2 : Constant  Value=-285.84E3
  Constant3 : Constant  Value=75.38
  Constant9 : Constant  Value=fc_cell_temp_ref
  Display : Display
      settings: Format=short  Decimation=12
  Product : Product  Inputs=2  Multiplication=Element-wise(.*)  SaturateOnIntegerOverflow=on
  Sum1 : Sum  Inputs=|++  SaturateOnIntegerOverflow=on
  Sum5 : Sum  Inputs=|+-  SaturateOnIntegerOverflow=on
  h_Wl [J/mol] : Outport  Port=1
  wires:
  Constant3/1 -> Product/1
  Sum5/1 -> Product/2
  Constant9/1 -> Sum5/2
  Constant12/1 -> Sum5/1
  Product/1 -> Sum1/2
  Constant2/1 -> Sum1/1
  Sum1/1 -> h_Wl [J/mol]/1, Display/1
